simulink library "LopesDevelopmentLibrary"  (R2015b)
settings: Solver=ode45  StartTime=0.0  StopTime=10.0  RelTol=1e-3
values from neighbouring files (symbols this model uses):
  d2r = @(d) d*(pi/180)    [LopesDevelopmentLibrary_LoadParameters.m]
  ts = LopesParams.ts    [LopesDevelopmentLibrary_LoadParameters.m]
undefined symbols (not defined in the file or in its folder): anyParameterChanged, DiscIntNeverNeededParam, gcbh, LAP, LHF, LKF, LopesParams, macaddr, mxpcnetworkconfig, mxpcrtudprx, mxpcrtudptx, patientParametersChanged, port, PX, PZ, RAP, RHF, RKF, SelectorLOPESInSize, StrideTime_s, Time
undefined symbols (not defined in the file): LopesParamsSendDataArrayLen
libraries: LopesDevelopmentLibrary x327, simulink x100, dspmtrx3 x49, xpciplib x6, xpcnetworkbufferlib x5, dspsigops x4, dspstat3 x3, xpcethernetlib x2, visionstatistics x2, xpcseriallib x2, LopesDevelopmentLibraryTest x1, nmc x1
(part 8 of 12)

== system LopesDevelopmentLibrary/BlocksForInternalUse/GaitGeneration/CalculateReferenceGait/CalculateAbductionLeft ==
  note: This version of the CalculateAbduction calculates
      | the derivatives analytically. At the end of the script there is a (commented)
      | Matlab script that calculates the derivatives using the symbolic toolbox. It shows analytically that
      | the velocity is calculated correctly, and the acceleration is too complex to solve for.
      | For the acceleration, I put in random numbers as input and compared the result of my own (optimized) equation
      | and the equation found by Matla Symbolic toolbox. They are equal, so that proves that my equations are all okay.
  note: This block calculates the abduction angle for one leg, given the actual pelvis position and the desired ankle position.
      | It does not take into account rotations of the pelvis, but the deviations from that are so small that that is not a problem.
  Parameters : Inport
  PelvisTZ : Inport  Port=2
  AnkleTZ : Inport  Port=3
  xHF : Inport  Port=4
  xKF : Inport  Port=5
  Bus Selector : BusSelector  OutputSignals=Patient.PelvisWidth_m,Patient.UpperLegLength_m,Patient.LowerLegLength_m
  Demux{,1..3} (4 alike) : Demux  Outputs=3
  MATLAB Function : MATLAB Function  TreatAsAtomicUnit=on
  Signal Conversion : SignalConversion
  isRight : Constant  Value=isRight
  Abduction : Outport
  dAbduction_dx : Outport  Port=2
  d2Abduction_dx2 : Outport  Port=3
  wires:
  isRight/1 -> MATLAB Function/1(isRight)
  PelvisTZ/1 -> Demux/1
  AnkleTZ/1 -> Demux1/1
  xHF/1 -> Demux2/1
  xKF/1 -> Demux3/1
  Parameters/1 -> Bus Selector/1
  Bus Selector/1 -> MATLAB Function/14(w_pelvis)  "<PelvisWidth_m>"
  Bus Selector/2 -> MATLAB Function/15(l_upper)  "<UpperLegLength_m>"
  Bus Selector/3 -> MATLAB Function/16(l_lower)  "<LowerLegLength_m>"
  MATLAB Function/1(Abduction) -> Signal Conversion/1
  MATLAB Function/2(dAbductiondx) -> dAbduction_dx/1
  MATLAB Function/3(ddAbductiondx) -> d2Abduction_dx2/1
  Signal Conversion/1 -> Abduction/1
  Demux/2 -> MATLAB Function/3(dPelvisTZdx)
  Demux/3 -> MATLAB Function/4(ddPelvisTZdx)
  Demux/1 -> MATLAB Function/2(PelvisTZ)
  Demux1/2 -> MATLAB Function/6(dAnkleTZdx)
  Demux1/1 -> MATLAB Function/5(AnkleTZ)
  Demux1/3 -> MATLAB Function/7(ddAnkleTZdx)
  Demux2/2 -> MATLAB Function/9(dxHFdx)
  Demux2/3 -> MATLAB Function/10(ddxHFdx)
  Demux2/1 -> MATLAB Function/8(xHF)
  Demux3/3 -> MATLAB Function/13(ddxKFdx)
  Demux3/1 -> MATLAB Function/11(xKF)
  Demux3/2 -> MATLAB Function/12(dxKFdx)

== system LopesDevelopmentLibrary/BlocksForInternalUse/GaitGeneration/CalculateReferenceGait/CalculateAbductionRight ==
  note: This block calculates the abduction angle for one leg, given the actual pelvis position and the desired ankle position.
      | It does not take into account rotations of the pelvis, but the deviations from that are so small that that is not a problem.
  note: This version of the CalculateAbduction calculates
      | the derivatives analytically. At the end of the script there is a (commented)
      | Matlab script that calculates the derivatives using the symbolic toolbox. It shows analytically that
      | the velocity is calculated correctly, and the acceleration is too complex to solve for.
      | For the acceleration, I put in random numbers as input and compared the result of my own (optimized) equation
      | and the equation found by Matla Symbolic toolbox. They are equal, so that proves that my equations are all okay.
  Parameters : Inport
  PelvisTZ : Inport  Port=2
  AnkleTZ : Inport  Port=3
  xHF : Inport  Port=4
  xKF : Inport  Port=5
  Bus Selector : BusSelector  OutputSignals=Patient.PelvisWidth_m,Patient.UpperLegLength_m,Patient.LowerLegLength_m
  Demux{,1..3} (4 alike) : Demux  Outputs=3
  MATLAB Function : MATLAB Function  TreatAsAtomicUnit=on
  Signal Conversion : SignalConversion
  isRight : Constant  Value=isRight
  Abduction : Outport
  dAbduction_dx : Outport  Port=2
  d2Abduction_dx2 : Outport  Port=3
  wires:
  Demux3/2 -> MATLAB Function/12(dxKFdx)
  Demux3/1 -> MATLAB Function/11(xKF)
  Demux3/3 -> MATLAB Function/13(ddxKFdx)
  Demux2/1 -> MATLAB Function/8(xHF)
  Demux2/3 -> MATLAB Function/10(ddxHFdx)
  Demux2/2 -> MATLAB Function/9(dxHFdx)
  Demux1/3 -> MATLAB Function/7(ddAnkleTZdx)
  Demux1/1 -> MATLAB Function/5(AnkleTZ)
  Demux1/2 -> MATLAB Function/6(dAnkleTZdx)
  Demux/1 -> MATLAB Function/2(PelvisTZ)
  Demux/3 -> MATLAB Function/4(ddPelvisTZdx)
  Demux/2 -> MATLAB Function/3(dPelvisTZdx)
  Signal Conversion/1 -> Abduction/1
  MATLAB Function/3(ddAbductiondx) -> d2Abduction_dx2/1
  MATLAB Function/2(dAbductiondx) -> dAbduction_dx/1
  MATLAB Function/1(Abduction) -> Signal Conversion/1
  Bus Selector/3 -> MATLAB Function/16(l_lower)  "<LowerLegLength_m>"
  Bus Selector/2 -> MATLAB Function/15(l_upper)  "<UpperLegLength_m>"
  Bus Selector/1 -> MATLAB Function/14(w_pelvis)  "<PelvisWidth_m>"
  Parameters/1 -> Bus Selector/1
  xKF/1 -> Demux3/1
  xHF/1 -> Demux2/1
  AnkleTZ/1 -> Demux1/1
  PelvisTZ/1 -> Demux/1
  isRight/1 -> MATLAB Function/1(isRight)

== system LopesDevelopmentLibrary/BlocksForInternalUse/GaitGeneration/CalculateReferenceGait/FirstDerivativeWrtTime ==
  dydx : Inport
  dtdx : Inport  Port=2
  Divide : Product  Inputs=*/
  dydt : Outport
  wires:
  Divide/1 -> dydt/1
  dydx/1 -> Divide/1
  dtdx/1 -> Divide/2

== system LopesDevelopmentLibrary/BlocksForInternalUse/GaitGeneration/CalculateReferenceGait/SecondDerivativeWrtTime ==
  ddydx : Inport
  dtdx : Inport  Port=2
  Divide1 : Product  Inputs=*/
  Math Function : Math  Operator=square  SaturateOnIntegerOverflow=on
  ddydt : Outport
  wires:
  dtdx/1 -> Math Function/1
  Math Function/1 -> Divide1/2
  ddydx/1 -> Divide1/1
  Divide1/1 -> ddydt/1

== system LopesDevelopmentLibrary/BlocksForInternalUse/GaitGeneration/CalculateReferenceGait/Unactuated DOFS ==

== system LopesDevelopmentLibrary/BlocksForInternalUse/GaitGenerationStartStop/ExtraKeyPoints /LeftAnklePF ==
  parameters : Inport
  SetVelocity : Inport  Port=2
  Bus Creator4 : BusCreator  Inputs=2
  Bus Selector : BusSelector  OutputSignals=General.WalkingVelocity_m_s,Patient.BodyLength_m
  RegressionData : Constant  Value=LopesParams.GaitDataStartLeft.LAP
  RegressionData2KeyEvents : LopesDevelopmentLibrary/BlocksForInternalUse/GaitGeneration/RegressionData2KeyEvents
  Switch : Switch  Criteria=u2 > Threshold
  KeyEvents : Outport
  wires:
  Switch/1 -> Bus Creator4/1  "WalkingVelocity_m_s"
  SetVelocity/1 -> Switch/1, Switch/2
  Bus Selector/1 -> Switch/3  "<WalkingVelocity_m_s>"
  Bus Selector/2 -> Bus Creator4/2  "<BodyLength_m>"
  Bus Creator4/1 -> RegressionData2KeyEvents/2
  parameters/1 -> Bus Selector/1
  RegressionData/1 -> RegressionData2KeyEvents/1
  RegressionData2KeyEvents/1 -> KeyEvents/1

== system LopesDevelopmentLibrary/BlocksForInternalUse/GaitGenerationStartStop/ExtraKeyPoints /LeftHipFlexion ==
  parameters : Inport
  SetVelocity : Inport  Port=2
  Bus Creator4 : BusCreator  Inputs=2
  Bus Selector : BusSelector  OutputSignals=General.WalkingVelocity_m_s,Patient.BodyLength_m
  RegressionData : Constant  Value=LopesParams.GaitDataStartLeft.LHF
  RegressionData2KeyEvents : LopesDevelopmentLibrary/BlocksForInternalUse/GaitGeneration/RegressionData2KeyEvents
  Switch : Switch  Criteria=u2 > Threshold
  KeyEvents : Outport
  wires:
  RegressionData2KeyEvents/1 -> KeyEvents/1
  parameters/1 -> Bus Selector/1
  RegressionData/1 -> RegressionData2KeyEvents/1
  Bus Creator4/1 -> RegressionData2KeyEvents/2
  Bus Selector/2 -> Bus Creator4/2  "<BodyLength_m>"
  Bus Selector/1 -> Switch/3  "<WalkingVelocity_m_s>"
  SetVelocity/1 -> Switch/2, Switch/1
  Switch/1 -> Bus Creator4/1  "WalkingVelocity_m_s"

== system LopesDevelopmentLibrary/BlocksForInternalUse/GaitGenerationStartStop/ExtraKeyPoints /LeftKneeFlexion ==
  parameters : Inport
  SetVelocity : Inport  Port=2
  Bus Creator4 : BusCreator  Inputs=2
  Bus Selector : BusSelector  OutputSignals=General.WalkingVelocity_m_s,Patient.BodyLength_m
  RegressionData : Constant  Value=LopesParams.GaitDataStartLeft.LKF
  RegressionData2KeyEvents : LopesDevelopmentLibrary/BlocksForInternalUse/GaitGeneration/RegressionData2KeyEvents
  Switch : Switch  Criteria=u2 > Threshold
  KeyEvents : Outport
  wires:
  RegressionData2KeyEvents/1 -> KeyEvents/1
  RegressionData/1 -> RegressionData2KeyEvents/1
  parameters/1 -> Bus Selector/1
  Bus Creator4/1 -> RegressionData2KeyEvents/2
  Bus Selector/2 -> Bus Creator4/2  "<BodyLength_m>"
  Bus Selector/1 -> Switch/3  "<WalkingVelocity_m_s>"
  SetVelocity/1 -> Switch/2, Switch/1
  Switch/1 -> Bus Creator4/1  "WalkingVelocity_m_s"

== system LopesDevelopmentLibrary/BlocksForInternalUse/GaitGenerationStartStop/ExtraKeyPoints /PelvisTPX ==
  parameters : Inport
  SetVelocity : Inport  Port=2
  Bus Creator4 : BusCreator  Inputs=2
  Bus Selector : BusSelector  OutputSignals=General.WalkingVelocity_m_s,Patient.BodyLength_m
  RegressionData : Constant  Value=LopesParams.GaitDataStartLeft.PX
  RegressionData2KeyEvents : LopesDevelopmentLibrary/BlocksForInternalUse/GaitGeneration/RegressionData2KeyEvents
  Switch : Switch  Criteria=u2 > Threshold
  KeyEvents : Outport
  wires:
  Switch/1 -> Bus Creator4/1  "WalkingVelocity_m_s"
  SetVelocity/1 -> Switch/1, Switch/2
  Bus Selector/1 -> Switch/3  "<WalkingVelocity_m_s>"
  Bus Selector/2 -> Bus Creator4/2  "<BodyLength_m>"
  Bus Creator4/1 -> RegressionData2KeyEvents/2
  RegressionData/1 -> RegressionData2KeyEvents/1
  parameters/1 -> Bus Selector/1
  RegressionData2KeyEvents/1 -> KeyEvents/1

== system LopesDevelopmentLibrary/BlocksForInternalUse/GaitGenerationStartStop/ExtraKeyPoints /PelvisTPZ ==
  parameters : Inport
  SetVelocity : Inport  Port=2
  Bus Creator4 : BusCreator  Inputs=2
  Bus Selector : BusSelector  OutputSignals=General.WalkingVelocity_m_s,Patient.BodyLength_m
  RegressionData : Constant  Value=LopesParams.GaitDataStartLeft.PZ
  RegressionData2KeyEvents : LopesDevelopmentLibrary/BlocksForInternalUse/GaitGeneration/RegressionData2KeyEvents
  Switch : Switch  Criteria=u2 > Threshold
  KeyEvents : Outport
  wires:
  Switch/1 -> Bus Creator4/1  "WalkingVelocity_m_s"
  SetVelocity/1 -> Switch/1, Switch/2
  Bus Selector/1 -> Switch/3  "<WalkingVelocity_m_s>"
  Bus Selector/2 -> Bus Creator4/2  "<BodyLength_m>"
  Bus Creator4/1 -> RegressionData2KeyEvents/2
  RegressionData/1 -> RegressionData2KeyEvents/1
  parameters/1 -> Bus Selector/1
  RegressionData2KeyEvents/1 -> KeyEvents/1

== system LopesDevelopmentLibrary/BlocksForInternalUse/GaitGenerationStartStop/ExtraKeyPoints /RightAnklePF ==
  parameters : Inport
  SetVelocity : Inport  Port=2
  Bus Creator4 : BusCreator  Inputs=2
  Bus Selector : BusSelector  OutputSignals=General.WalkingVelocity_m_s,Patient.BodyLength_m
  RegressionData : Constant  Value=LopesParams.GaitDataStartLeft.RAP
  RegressionData2KeyEvents : LopesDevelopmentLibrary/BlocksForInternalUse/GaitGeneration/RegressionData2KeyEvents
  Switch : Switch  Criteria=u2 > Threshold
  KeyEvents : Outport
  wires:
  Switch/1 -> Bus Creator4/1  "WalkingVelocity_m_s"
  SetVelocity/1 -> Switch/1, Switch/2
  Bus Selector/1 -> Switch/3  "<WalkingVelocity_m_s>"
  Bus Selector/2 -> Bus Creator4/2  "<BodyLength_m>"
  Bus Creator4/1 -> RegressionData2KeyEvents/2
  parameters/1 -> Bus Selector/1
  RegressionData/1 -> RegressionData2KeyEvents/1
  RegressionData2KeyEvents/1 -> KeyEvents/1

== system LopesDevelopmentLibrary/BlocksForInternalUse/GaitGenerationStartStop/ExtraKeyPoints /RightHipFlexion ==
  parameters : Inport
  SetVelocity : Inport  Port=2
  Bus Creator4 : BusCreator  Inputs=2
  Bus Selector : BusSelector  OutputSignals=General.WalkingVelocity_m_s,Patient.BodyLength_m
  RegressionData : Constant  Value=LopesParams.GaitDataStartLeft.RHF
  RegressionData2KeyEvents : LopesDevelopmentLibrary/BlocksForInternalUse/GaitGeneration/RegressionData2KeyEvents
  Switch : Switch  Criteria=u2 > Threshold
  KeyEvents : Outport
  wires:
  RegressionData/1 -> RegressionData2KeyEvents/1
  RegressionData2KeyEvents/1 -> KeyEvents/1
  parameters/1 -> Bus Selector/1
  Bus Creator4/1 -> RegressionData2KeyEvents/2
  Bus Selector/2 -> Bus Creator4/2  "<BodyLength_m>"
  Bus Selector/1 -> Switch/3  "<WalkingVelocity_m_s>"
  SetVelocity/1 -> Switch/2, Switch/1
  Switch/1 -> Bus Creator4/1  "WalkingVelocity_m_s"

== system LopesDevelopmentLibrary/BlocksForInternalUse/GaitGenerationStartStop/ExtraKeyPoints /RightKneeFlexion ==
  parameters : Inport
  SetVelocity : Inport  Port=2
  Bus Creator4 : BusCreator  Inputs=2
  Bus Selector : BusSelector  OutputSignals=General.WalkingVelocity_m_s,Patient.BodyLength_m
  RegressionData : Constant  Value=LopesParams.GaitDataStartLeft.RKF
  RegressionData2KeyEvents : LopesDevelopmentLibrary/BlocksForInternalUse/GaitGeneration/RegressionData2KeyEvents
  Switch : Switch  Criteria=u2 > Threshold
  KeyEvents : Outport
  wires:
  RegressionData2KeyEvents/1 -> KeyEvents/1
  RegressionData/1 -> RegressionData2KeyEvents/1
  parameters/1 -> Bus Selector/1
  Bus Creator4/1 -> RegressionData2KeyEvents/2
  Bus Selector/2 -> Bus Creator4/2  "<BodyLength_m>"
  Bus Selector/1 -> Switch/3  "<WalkingVelocity_m_s>"
  SetVelocity/1 -> Switch/2, Switch/1
  Switch/1 -> Bus Creator4/1  "WalkingVelocity_m_s"

== system LopesDevelopmentLibrary/BlocksForInternalUse/LLC Communication/LLC Network Configuration/Variant Network Init ==
  note: 1) Only subsystems can be added as variant choices at this level
      | 2) Blocks cannot be connected at this level as connectivity is
      | automatically determined at simulation, based on the active variant
  note: I did not remove the inputs/outputs because that makes Matlab fail...
  Dummy_in : Inport
  Init_NonRT_UDP : Subsystem  VariantControl=LopesVariant_Non_RT
  Init_RT_2012b : Subsystem  VariantControl=LopesVariant_RT_2012b
  Init_RT_2014b : Subsystem  VariantControl=LopesVariant_RT_2014b
  Init_RT_2015b : Subsystem  VariantControl=LopesVariant_RT_2015b
  Dummy_out : Outport

== system LopesDevelopmentLibrary/BlocksForInternalUse/LLC Communication/LLCReceiveUDP/Debug ==

== system LopesDevelopmentLibrary/BlocksForInternalUse/LLC Communication/LLCReceiveUDP/UDPReceiveVariantChannel ==
  note: 1) Add Subsystem or Model blocks as valid variant choices.
      | 2) You cannot connect blocks at this level. At simulation, connectivity is automatically
      | determined, based on the active variant and port name matching.
  Dummy_in : Inport
  Receive_Non_RT : Subsystem  VariantControl=LopesVariant_Non_RT
  Receive_RT_2015b : Subsystem  VariantControl=LopesVariant_RT_2015b
  Receive_RT_R2012b : Subsystem  VariantControl=LopesVariant_RT_2012b
  Receive_RT_R2014b : Subsystem  VariantControl=LopesVariant_RT_2014b
  RecvData : Outport
  RecvLen : Outport  Port=2

== system LopesDevelopmentLibrary/BlocksForInternalUse/LLC Communication/LLCSendUDP/Debug ==

== system LopesDevelopmentLibrary/BlocksForInternalUse/LLC Communication/LLCSendUDP/UDPSendVariant ==
  Data : Inport
  Len : Inport  Port=2
  Enable : EnablePort
  Terminator : Terminator
  UDPSendVariantChannel : Subsystem  Variant=on
  wires:
  Data/1 -> UDPSendVariantChannel/1(SendData)
  Len/1 -> UDPSendVariantChannel/2(SendLen)
  UDPSendVariantChannel/1(Dummy_out) -> Terminator/1

== system LopesDevelopmentLibrary/BlocksForInternalUse/LLC Communication/UDP_Blocks/Network Configuration_RT_2012b  ==
  "ARP Init " : S-Function  Priority=0  FunctionName=xpcdebugarpinit  Parameters=Stats, Interface, IpAddress, SubnetMask, Gateway, EthernetId, Flags, BlockId, Retry, Timeout, Expiration, StaticAddressListIp, StaticAddressListMac, DiscoveryList, MulticastList, SampleTime  SFunctionDeploymentMode=off  EnableBusSupport=off  mask(arpinit){Interface=0, IpAddress=IpAddress, SubnetMask=SubnetMask, Gateway=Gateway, EthernetId=1, BlockId=0, SampleTime=-1, Flags=hex2dec('00000697'), Stats=off, Retry=5, Timeout=20, Expiration=20*60, StaticAddressListIp=[], StaticAddressListMac=[], DiscoveryList=[], MulticastList=[]}
      mask prompts: IpAddress "IP Address"; SubnetMask "Subnet Mask"; EthernetId "Ethernet ID"; BlockId "Block ID"; SampleTime "Sample Time"; Stats "Statistics Port"; StaticAddressListIp "[Static IP]"; StaticAddressListMac "[Static MAC]"; DiscoveryList "[Discovery IP]"; MulticastList "[Multicast IP]"
      mask help: ARP Init
      mask init:
      | xpclinklib('xpciplib');
      mask Help: web('arpdebug.htm',  '-helpbrowser');
      mask Display: disp('ARP Init');
  "Buffer Mngmt " : S-Function  Priority=-1  FunctionName=xpcnb  Parameters=pool_sizes, SampleTime, ShowTune  SFunctionDeploymentMode=off  EnableBusSupport=off  mask(xpcnbinit){SampleTime=-1, PoolSizes=[100 10 10 200], ShowTune=off}
      mask prompts: SampleTime "Sample time:"; PoolSizes "Buffer pool sizes (256, 512, 1024, 2048):"; ShowTune "Display tuning information"
      mask help: Network Buffer Initialization
      mask init:
      | [MaskDisplay, pool_sizes] = mxpcnbinit(2, PoolSizes);
      | 
      | set_param(gcb, 'MaskDisplay', MaskDisplay);
      mask Help: eval('xpcdoc(''NB_Init'')');
      mask Display: disp('Network Buffer\nManagement');
  "Ethernet Init " : S-Function  Priority=-1  FunctionName=xpcetherinit  Parameters="ID, Driver, Bus, Slot, VendorID, DeviceID, AddressSource, mac, TxSA, RxPromiscuous, RxBad, RxShort, MaxMTU, TxThreshold, TxBuffers, RxBuffers, ShowTune, numMulti, multicast,   NumRxBlks, SampleTime"  SFunctionDeploymentMode=off  EnableBusSupport=off  mask(xpcetherinit){ID=1, Driver=EthDrv, Bus=PciBus, Slot=PciSlot, SampleTime=-1, AddressSource=EEPROM, MAC=macaddr('00:00:00:00:00:00'), TxSA=off, RxPromiscuous=off, Multicast={}, RxBad=off, RxShort=off, MaxMTU=1518, TxThreshold=224, TxBuffers=128, RxBuffers=64, ShowTune=off, NumRxBlks=1}
      mask prompts: ID "Device ID:"; Bus "PCI bus:"; Slot "PCI slot:"; SampleTime "Sample time:"; AddressSource "Address source:"; TxSA "Tx source address from model"; RxPromiscuous "Rx promiscuous"; Multicast "Multicast address list:"; RxBad "Rx bad frames"; RxShort "Rx short frames"; MaxMTU "Max MTU:"; TxThreshold "Tx threshold:"; TxBuffers "Tx buffers:"; RxBuffers "Rx buffers:"; ShowTune "Display tuning information"; NumRxBlks "num rx blocks"
      mask help: Ethernet Initialization
      mask init:
      | VendorID = -1;
      | DeviceID = -1;
      | 
      | [MaskDisplay, VendorID, DeviceID, mac, numMulti, multicast] = mxpcetherinit(2, ID, Driver, Bus, Slot, MAC, Multicast);
      | 
      | set_param(gcb, 'MaskDisplay', MaskDisplay);
      mask Help: eval('xpcdoc(''Ether_Init'')');
      mask TypeOptions ID: 1 | 2 | 3 | 4 | 5 | 6 | 7 | 8
      mask TypeOptions AddressSource: EEPROM | Specify
      mask Callback AddressSource:
      | enables = get_param(gcb, 'MaskVisibilities');
      | if strcmp('Specify', get_param(gcb, 'AddressSource'))
      |     enables{strmatch('MAC',fieldnames(get_param(gcb,'DialogParameters')))} = 'on';
      | else
      |     enables{strmatch('MAC',fieldnames(get_param(gcb,'DialogParameters')))} = 'off';
      | end
      | set_param(gcb, 'MaskVisibilities', enables);
      mask Display: disp('Ethernet\nInitialization\nbus: 1 slot: 0\nId: 1\nIntel Gigabit');
  "IP Init " : S-Function  Priority=1  FunctionName=xpcdebugipinit  Parameters=Stats, Group, ArpId, IpAddress, SubnetMask, DefaultGateway, DefaultInterface, Flags, ToS, StartingId, TTL, SampleTime  SFunctionDeploymentMode=off  EnableBusSupport=off  mask(ipinit){Group=0, ArpId=[0], IpAddress=[IpAddress], SubnetMask=[SubnetMask], DefaultGateway=Gateway, DefaultInterface=0, SampleTime=-1, Flags=hex2dec('00000005'), ToS=hex2dec('00'), StartingId=10000, TTL=64, Stats=off}
      mask prompts: ArpId "[ARP ID]"; IpAddress "[IP Address]"; SubnetMask "[Subnet Mask]"; DefaultGateway "Default Gateway"; DefaultInterface "Default Interface"; SampleTime "Sample Time"; StartingId "Starting Id"; Stats "Statistics Port"
      mask help: IP Init
      mask init:
      | xpclinklib('xpciplib');
      mask Help: web('ipdebug.htm',  '-helpbrowser');
      mask Display: disp('IP Init');
  "UDP Init " : S-Function  Priority=2  FunctionName=xpcdebugudpinit  Parameters=Stats, Group, StartingPort, Flags, SampleTime  SFunctionDeploymentMode=off  EnableBusSupport=off  mask(udpinit){Group=0, StartingPort=10000, Flags=hex2dec('00000001'), SampleTime=-1, Stats=off}
      mask prompts: StartingPort "Starting Port"; SampleTime "Sample Time"; Stats "Statistics Port"
      mask help: UDP Init
      mask init:
      | xpclinklib('xpciplib');
      mask Help: web('udpdebug.htm',  '-helpbrowser');
      mask Display: disp('UDP Init');

== system LopesDevelopmentLibrary/BlocksForInternalUse/LLC Communication/UDP_Blocks/Network Configuration_RT_2014b  ==
  "ARP Init " : S-Function  Priority=0  FunctionName=xpcdebugarpinit  Parameters=Stats, Interface, IpAddress, SubnetMask, Gateway, EthernetId, Flags, BlockId, Retry, Timeout, Expiration, StaticAddressListIp, StaticAddressListMac, DiscoveryList, MulticastList, SampleTime  SFunctionDeploymentMode=off  EnableBusSupport=off  mask(arpinit){Interface=udpID, IpAddress=IpAddress, SubnetMask=SubnetMask, Gateway=Gateway, EthernetId=ID, BlockId=0, SampleTime=-1, Flags=hex2dec('00000697'), Stats=off, Retry=5, Timeout=20, Expiration=20*60, StaticAddressListIp=[], StaticAddressListMac=[], DiscoveryList=[], MulticastList=[]}
      mask prompts: IpAddress "IP Address"; SubnetMask "Subnet Mask"; EthernetId "Ethernet ID"; BlockId "Block ID"; SampleTime "Sample Time"; Stats "Statistics Port"; StaticAddressListIp "[Static IP]"; StaticAddressListMac "[Static MAC]"; DiscoveryList "[Discovery IP]"; MulticastList "[Multicast IP]"
      mask help: ARP Init
      mask init:
      | xpclinklib('xpciplib');
      mask Help: web('arpdebug.htm',  '-helpbrowser');
      mask Display: disp('ARP Init');
  "Buffer Mngmt " : xpcnetworkbufferlib/Buffer Mngmt   Priority=-1  SampleTime=-1  PoolSizes=[100 10 10 200]  ShowTune=off
  "Ethernet Init " : xpcethernetlib/Ethernet Init   Priority=-1  ID=1  Driver=Intel Gigabit  Bus=PciBus  Slot=PciSlot  SampleTime=-1  AddressSource=EEPROM  MAC=macaddr('00:00:00:00:00:00')  TxSA=off  RxPromiscuous=off  Multicast={}  RxBad=off  RxShort=off  MaxMTU=1518  TxThreshold=224  TxBuffers=128  RxBuffers=64  ShowTune=off  NumRxBlks=1
  "IP Init " : S-Function  Priority=1  FunctionName=xpcdebugipinit  Parameters=Stats, Group, ArpId, IpAddress, SubnetMask, DefaultGateway, DefaultInterface, Flags, ToS, StartingId, TTL, SampleTime  SFunctionDeploymentMode=off  EnableBusSupport=off  mask(ipinit){Group=udpID, ArpId=[udpID], IpAddress=[IpAddress], SubnetMask=[SubnetMask], DefaultGateway=Gateway, DefaultInterface=0, SampleTime=-1, Flags=hex2dec('00000005'), ToS=hex2dec('00'), StartingId=10000, TTL=64, Stats=off}
      mask prompts: ArpId "[ARP ID]"; IpAddress "[IP Address]"; SubnetMask "[Subnet Mask]"; DefaultGateway "Default Gateway"; DefaultInterface "Default Interface"; SampleTime "Sample Time"; StartingId "Starting Id"; Stats "Statistics Port"
      mask help: IP Init
      mask init:
      | xpclinklib('xpciplib');
      mask Help: web('ipdebug.htm',  '-helpbrowser');
      mask Display: disp('IP Init');
  "UDP Init " : S-Function  Priority=2  FunctionName=xpcdebugudpinit  Parameters=Stats, Group, StartingPort, Flags, SampleTime  SFunctionDeploymentMode=off  EnableBusSupport=off  mask(udpinit){Group=udpID, StartingPort=10000, Flags=hex2dec('00000001'), SampleTime=-1, Stats=off}
      mask prompts: StartingPort "Starting Port"; SampleTime "Sample Time"; Stats "Statistics Port"
      mask help: UDP Init
      mask init:
      | xpclinklib('xpciplib');
      mask Help: web('udpdebug.htm',  '-helpbrowser');
      mask Display: disp('UDP Init');

== system LopesDevelopmentLibrary/BlocksForInternalUse/LLC Communication/UDP_Blocks/Network Configuration_RT_2015b ==
  "ARP Init " : S-Function  Priority=0  FunctionName=xpcdebugarpinit  Parameters=Stats, Interface, IpAddress, SubnetMask, Gateway, EthernetId, Flags, BlockId, Retry, Timeout, Expiration, StaticAddressListIp, StaticAddressListMac, DiscoveryList, MulticastList, SampleTime  SFunctionDeploymentMode=off  EnableBusSupport=off  mask(arpinit){Interface=udpID, IpAddress=IpAddress, SubnetMask=SubnetMask, Gateway=Gateway, EthernetId=ID, BlockId=0, SampleTime=-1, Flags=hex2dec('00000697'), Stats=off, Retry=5, Timeout=20, Expiration=20*60, StaticAddressListIp=[], StaticAddressListMac=[], DiscoveryList=[], MulticastList=MulticastList}
      mask prompts: IpAddress "IP Address"; SubnetMask "Subnet Mask"; EthernetId "Ethernet ID"; BlockId "Block ID"; SampleTime "Sample Time"; Stats "Statistics Port"; StaticAddressListIp "[Static IP]"; StaticAddressListMac "[Static MAC]"; DiscoveryList "[Discovery IP]"; MulticastList "[Multicast IP]"
      mask help: ARP Init
      mask init:
      | xpclinklib('xpciplib');
      mask Help: web('arpdebug.htm',  '-helpbrowser');
      mask Display: disp('ARP Init');
  "Buffer Mngmt " : xpcnetworkbufferlib/Buffer Mngmt   Priority=-1  SampleTime=-1  PoolSizes=[100 10 10 200]  ShowTune=off
  "Ethernet Init " : xpcethernetlib/Ethernet Init   Priority=-1  ID=1  Driver=Intel Gigabit  Bus=PciBus  Slot=PciSlot  SampleTime=-1  AddressSource=EEPROM  MAC=macaddr('00:00:00:00:00:00')  TxSA=off  RxPromiscuous=off  Multicast=Multicast  RxBad=off  RxShort=off  MaxMTU=1518  TxThreshold=224  TxBuffers=128  RxBuffers=64  ShowTune=off  NumRxBlks=1
  "IP Init " : S-Function  Priority=1  FunctionName=xpcdebugipinit  Parameters=Stats, Group, ArpId, IpAddress, SubnetMask, DefaultGateway, DefaultInterface, Flags, ToS, StartingId, TTL, SampleTime  SFunctionDeploymentMode=off  EnableBusSupport=off  mask(ipinit){Group=udpID, ArpId=[udpID], IpAddress=[IpAddress], SubnetMask=[SubnetMask], DefaultGateway=Gateway, DefaultInterface=0, SampleTime=-1, Flags=hex2dec('00000005'), ToS=hex2dec('00'), StartingId=10000, TTL=64, Stats=off}
      mask prompts: ArpId "[ARP ID]"; IpAddress "[IP Address]"; SubnetMask "[Subnet Mask]"; DefaultGateway "Default Gateway"; DefaultInterface "Default Interface"; SampleTime "Sample Time"; StartingId "Starting Id"; Stats "Statistics Port"
      mask help: IP Init
      mask init:
      | xpclinklib('xpciplib');
      mask Help: web('ipdebug.htm',  '-helpbrowser');
      mask Display: disp('IP Init');
  "UDP Init " : S-Function  Priority=2  FunctionName=xpcdebugudpinit  Parameters=Stats, Group, StartingPort, Flags, SampleTime  SFunctionDeploymentMode=off  EnableBusSupport=off  mask(udpinit){Group=udpID, StartingPort=10000, Flags=hex2dec('00000001'), SampleTime=-1, Stats=off}
      mask prompts: StartingPort "Starting Port"; SampleTime "Sample Time"; Stats "Statistics Port"
      mask help: UDP Init
      mask init:
      | xpclinklib('xpciplib');
      mask Help: web('udpdebug.htm',  '-helpbrowser');
      mask Display: disp('UDP Init');

== system LopesDevelopmentLibrary/BlocksForInternalUse/LLC Communication/UDP_Blocks/Receive_RT_2012b  ==
  "Buffer " : S-Function  FunctionName=xpcnbbuffer  Parameters=chainSize, bufferSize, Threshold  SFunctionDeploymentMode=off  EnableBusSupport=off  mask(xpcnbbuffer){ChainSize=1, BufferSize=0, Threshold=0}
      mask prompts: ChainSize "Chain size:"; BufferSize "Buffer size:"
      mask help:
      | Network Buffer Buffering
      |
      | Chain size = inf --> No buffering, all packets passed through
      | Chain size = 0   --> Deletes all packets, none passed through
      | Chain size > 0   --> Passes through first "Chain size" packets
      | Chain size < 0   --> Passes through last "Chain size" packets
      |
      | Buffer size = inf --> All remaining packets are buffered, none are deleted
      | Buffer size = 0   --> No buffering, deletes all remaining packets
      | Buffer size > 0   --> Buffers remaining first "Buffer size" packets
      | Buffer size < 0   --> Buffers remaining last "Buffer size" packets
      |
      | Threshold = 0 --> No threshold
      | Threshold > 0 --> Delay passing through packets till threshold is met once
      | Threshold < 0 --> Passes through packets if "Threshold" packets are buffered
      mask init:
      | [MaskDisplay, chainSize, bufferSize] = mxpcnbbuffer(2, ChainSize, BufferSize, Threshold);
      | 
      | set_param(gcb, 'MaskDisplay', MaskDisplay);
      mask Help: helpview(fullfile(docroot, 'mapfiles', 'xpc.map'), 'NB_Buffer')
      mask Display: disp('NB\nBuffering\n\n');port_label('output', 1, '1');
  "Extract " : S-Function  FunctionName=xpcnbextract  Parameters=packetSize  SFunctionDeploymentMode=off  EnableBusSupport=off  mask(xpcnbextract){PacketSize=Receive3}
      mask prompts: PacketSize "Packet size (-1: inherit):"
      mask help: Network Buffer Extract
      mask init:
      | [packetSize] = mxpcnbextract(2,PacketSize);
      mask Help: helpview(fullfile(docroot, 'mapfiles', 'xpc.map'), 'NB_Extract')
      mask Display: disp('NB Extract\n');port_label('output', 2, 'length');
  Terminator : Terminator
  "UDP Consume " : S-Function  FunctionName=xpcudpconsume  Parameters=Group, VectorSize, SampleTime  SFunctionDeploymentMode=off  EnableBusSupport=off  mask(udpconsume){Group=0, VectorSize=0, SampleTime=Receive4}
      mask prompts: Group "IP Group"; VectorSize "Output port width:"; SampleTime "Sample time:"
      mask help: UDP Consume
      mask Help: helpview(fullfile(docroot, 'mapfiles', 'xpc.map'), 'RT_UDP_CONSUME')
      mask Display:
      | if VectorSize
      |     disp('UDP Consume\n\n\n\n\n\n\n');
      |     port_label('output', 1, 'Buffers');
      |     port_label('output', 2, 'Source IP Address');
      |     port_label('output', 3, 'Destination IP Address');
      |     port_label('output', 4, 'Local UDP Port');
      |     port_label('output', 5, 'Remote UDP Port');
      |     port_label('output', 6, 'Chain Size');
      | else
      |     disp('UDP Consume');
      |     port_label('output', 1, 'Buffers');
      |     port_label('output', 2, 'Chain Size');
      | end
  "UDP Rx " : S-Function  Priority=5  FunctionName=xpcudprx  Parameters=Group, SourceAddress, sip, LocalPort, lup, SampleTime  SFunctionDeploymentMode=off  EnableBusSupport=off  mask(udprx){Group=0, sip=Any, SourceAddress=Receive1, lup=Specify, LocalPort=Receive2, SampleTime=Receive4}
      mask prompts: Group "IP Group"; sip "Source IP Address"; SourceAddress "IP address to receive from (0.0.0.0 for accepting all):"; lup "Local UDP Port"; LocalPort "IP port to receive from:"; SampleTime "Sample time:"
      mask help: UDP Rx
      mask init:
      | if SourceAddress == 0
      |     sip = 3;
      | end
      | 
      | SourceAddress = ipaddr(SourceAddress);
      mask Help: helpview(fullfile(docroot, 'mapfiles', 'xpc.map'), 'RT_UDP_RX')
      mask TypeOptions sip: Specify | Port | Any
      mask TypeOptions lup: Specify | Port | Any
      mask Display: disp('UDP Rx');
  Out1 : Outport  OutDataTypeStr=uint8
  Out2 : Outport  Port=2  OutDataTypeStr=double
  wires:
  "UDP Consume "/2 -> Terminator/1
  "UDP Consume "/1 -> "Extract "/1
  "UDP Rx "/1 -> "Buffer "/1
  "Buffer "/1 -> "UDP Consume "/1
  "Extract "/1 -> Out1/1
  "Extract "/2 -> Out2/1

== system LopesDevelopmentLibrary/BlocksForInternalUse/LLC Communication/UDP_Blocks/Receive_RT_2014b  ==
  "Buffer " : S-Function  FunctionName=xpcnbbuffer  Parameters=chainSize, bufferSize, Threshold  SFunctionDeploymentMode=off  EnableBusSupport=off  mask(xpcnbbuffer){ChainSize=1, BufferSize=0, Threshold=0}
      mask prompts: ChainSize "Chain size:"; BufferSize "Buffer size:"
      mask help:
      | Network Buffer Buffering
      |
      | Chain size = inf --> No buffering, all packets passed through
      | Chain size = 0   --> Deletes all packets, none passed through
      | Chain size > 0   --> Passes through first "Chain size" packets
      | Chain size < 0   --> Passes through last "Chain size" packets
      |
      | Buffer size = inf --> All remaining packets are buffered, none are deleted
      | Buffer size = 0   --> No buffering, deletes all remaining packets
      | Buffer size > 0   --> Buffers remaining first "Buffer size" packets
      | Buffer size < 0   --> Buffers remaining last "Buffer size" packets
      |
      | Threshold = 0 --> No threshold
      | Threshold > 0 --> Delay passing through packets till threshold is met once
      | Threshold < 0 --> Passes through packets if "Threshold" packets are buffered
      mask init:
      | [MaskDisplay, chainSize, bufferSize] = mxpcnbbuffer(2, ChainSize, BufferSize, Threshold);
      | 
      | set_param(gcb, 'MaskDisplay', MaskDisplay);
      mask Help: helpview(fullfile(docroot, 'mapfiles', 'xpc.map'), 'NB_Buffer')
      mask Display: disp('NB\nBuffering\n\n');port_label('output', 1, '1');
  "Extract " : S-Function  FunctionName=xpcnbextract  Parameters=packetSize  SFunctionDeploymentMode=off  EnableBusSupport=off  mask(xpcnbextract){PacketSize=Receive3}
      mask prompts: PacketSize "Packet size (-1: inherit):"
      mask help: Network Buffer Extract
      mask init:
      | [packetSize] = mxpcnbextract(2,PacketSize);
      mask Help: helpview(fullfile(docroot, 'mapfiles', 'xpc.map'), 'NB_Extract')
      mask Display: disp('NB Extract\n');port_label('output', 2, 'length');
  Terminator : Terminator
  "UDP Consume " : S-Function  FunctionName=xpcudpconsume  Parameters=Group, VectorSize, SampleTime  SFunctionDeploymentMode=off  EnableBusSupport=off  mask(udpconsume){Group=udpID, VectorSize=0, SampleTime=Receive4}
      mask prompts: Group "IP Group"; VectorSize "Output port width:"; SampleTime "Sample time:"
      mask help: UDP Consume
      mask Help: helpview(fullfile(docroot, 'mapfiles', 'xpc.map'), 'RT_UDP_CONSUME')
      mask Display:
      | if VectorSize
      |     disp('UDP Consume\n\n\n\n\n\n\n');
      |     port_label('output', 1, 'Buffers');
      |     port_label('output', 2, 'Source IP Address');
      |     port_label('output', 3, 'Destination IP Address');
      |     port_label('output', 4, 'Local UDP Port');
      |     port_label('output', 5, 'Remote UDP Port');
      |     port_label('output', 6, 'Chain Size');
      | else
      |     disp('UDP Consume');
      |     port_label('output', 1, 'Buffers');
      |     port_label('output', 2, 'Chain Size');
      | end
  "UDP Rx " : S-Function  Priority=5  FunctionName=xpcudprx  Parameters=Group, SourceAddress, sip, LocalPort, lup, SampleTime  SFunctionDeploymentMode=off  EnableBusSupport=off  mask(udprx){Group=udpID, sip=Any, SourceAddress=Receive1, lup=Specify, LocalPort=Receive2, SampleTime=Receive4}
      mask prompts: Group "IP Group"; sip "Source IP Address"; SourceAddress "IP address to receive from (0.0.0.0 for accepting all):"; lup "Local UDP Port"; LocalPort "IP port to receive from:"; SampleTime "Sample time:"
      mask help: UDP Rx
      mask init:
      | if SourceAddress == 0
      |     sip = 3;
      | else
      |     sip = 1;
      | end
      mask Help: helpview(fullfile(docroot, 'mapfiles', 'xpc.map'), 'RT_UDP_RX')
      mask TypeOptions sip: Specify | Port | Any
      mask TypeOptions lup: Specify | Port | Any
      mask Display: disp('UDP Rx');
  Out1 : Outport  OutDataTypeStr=uint8
  Out2 : Outport  Port=2  OutDataTypeStr=double
  wires:
  "UDP Consume "/2 -> Terminator/1
  "UDP Consume "/1 -> "Extract "/1
  "UDP Rx "/1 -> "Buffer "/1
  "Buffer "/1 -> "UDP Consume "/1
  "Extract "/1 -> Out1/1
  "Extract "/2 -> Out2/1

== system LopesDevelopmentLibrary/BlocksForInternalUse/LLC Communication/UDP_Blocks/Receive_RT_2015b ==
  Buffer 1 : xpcnetworkbufferlib/Manage   ChainSize=1  BufferSize=0  Threshold=0
  Extract 1 : xpcnetworkbufferlib/Extract   PacketSize=Receive3
  Terminator : Terminator
  UDP Consume 1 : xpciplib/UDP Consume   Group=udpID  VectorSize=0  SampleTime=Receive4
  UDP Rx 1 : xpciplib/UDP Rx   Priority=5  Group=udpID  sip=Any  SourceAddress=Receive1  lup=Specify  LocalPort=Receive2  SampleTime=Receive4
  Out1 : Outport  OutDataTypeStr=uint8
  Out2 : Outport  Port=2  OutDataTypeStr=double
  wires:
  UDP Consume 1/2 -> Terminator/1
  UDP Consume 1/1 -> Extract 1/1
  UDP Rx 1/1 -> Buffer 1/1
  Buffer 1/1 -> UDP Consume 1/1
  Extract 1/1 -> Out1/1
  Extract 1/2 -> Out2/1

== system LopesDevelopmentLibrary/BlocksForInternalUse/LLC Communication/UDP_Blocks/Send_RT_2012b ==
  In1 : Inport  OutDataTypeStr=uint8
  In2 : Inport  Port=2  OutDataTypeStr=double
  "Compose " : S-Function  FunctionName=xpcnbcompose  SFunctionDeploymentMode=off  EnableBusSupport=off  mask(xpcnbcompose){}
      mask help: Network Buffer Compose
      mask init:
      | mxpcnbcompose(2);
      mask Help: helpview(fullfile(docroot, 'mapfiles', 'xpc.map'), 'NB_Compose')
      mask Display: disp('NB Compose\n');port_label('input', 2, 'length');
  "UDP Produce " : S-Function  Priority=5  FunctionName=xpcudpproduce  Parameters=Group, SrcIp, sip, DstIp, dip, LocPort, lup, RemPort, rup, SampleTime  SFunctionDeploymentMode=off  EnableBusSupport=off  mask(udpproduce){Group=0, sip=Auto, SrcIp=0.0.0.0, dip=Specify, DstIp=Send1, rup=Specify, RemPort=Send2, lup=Auto, LocPort=Send3, SampleTime=Send4}
      mask prompts: Group "IP Group"; sip "Source IP Address"; SrcIp "Source IP Address"; dip "Destination IP Address"; DstIp "IP address to send to (255.255.255.255 for broadcast):"; rup "Remote UDP Port"; RemPort "Remote IP port to send to:"; lup "Local UDP Port"; LocPort "Use the following local IP port (-1 for automatic assignment):"; SampleTime "Sample time:"
      mask help: UDP Produce
      mask init:
      | if LocPort == -1
      |     lup = 3;
      | end
      | 
      | SrcIp = ipaddr(SrcIp);
      | DstIp = ipaddr(DstIp);
      mask Help: helpview(fullfile(docroot, 'mapfiles', 'xpc.map'), 'RT_UDP_PRODUCE')
      mask TypeOptions sip: Specify | Port | Auto
      mask TypeOptions dip: Specify | Port
      mask TypeOptions rup: Specify | Port
      mask TypeOptions lup: Specify | Port | Auto
      mask Display: disp('UDP Produce');
  "UDP Tx " : xpciplib/UDP Tx   Priority=5  Group=0  TTL=-1  ToS=-1  SampleTime=Send4
  wires:
  "UDP Produce "/1 -> "UDP Tx "/1
  "Compose "/1 -> "UDP Produce "/1
  In1/1 -> "Compose "/1
  In2/1 -> "Compose "/2

== system LopesDevelopmentLibrary/BlocksForInternalUse/LLC Communication/UDP_Blocks/Send_RT_2014b ==
  In1 : Inport  OutDataTypeStr=uint8
  In2 : Inport  Port=2  OutDataTypeStr=double
  "Compose " : S-Function  FunctionName=xpcnbcompose  SFunctionDeploymentMode=off  EnableBusSupport=off  mask(xpcnbcompose){}
      mask help: Network Buffer Compose
      mask init:
      | mxpcnbcompose(2);
      mask Help: helpview(fullfile(docroot, 'mapfiles', 'xpc.map'), 'NB_Compose')
      mask Display: disp('NB Compose\n');port_label('input', 2, 'length');
  "UDP Produce " : S-Function  Priority=5  FunctionName=xpcudpproduce  Parameters=Group, SrcIp, sip, DstIp, dip, LocPort, lup, RemPort, rup, SampleTime  SFunctionDeploymentMode=off  EnableBusSupport=off  mask(udpproduce){Group=udpID, sip=Auto, SrcIp=0.0.0.0, dip=Specify, DstIp=Send1, rup=Specify, RemPort=Send2, lup=Auto, LocPort=Send3, SampleTime=Send4}
      mask prompts: Group "IP Group"; sip "Source IP Address"; SrcIp "Source IP Address"; dip "Destination IP Address"; DstIp "IP address to send to (255.255.255.255 for broadcast):"; rup "Remote UDP Port"; RemPort "Remote IP port to send to:"; lup "Local UDP Port"; LocPort "Use the following local IP port (-1 for automatic assignment):"; SampleTime "Sample time:"
      mask help: UDP Produce
      mask init:
      | if LocPort == -1
      |     lup = 3;
      | else
      |     lup = 1;
      | end
      | 
      | SrcIp = ipaddr(SrcIp);
      | DstIp = ipaddr(DstIp);
      mask Help: helpview(fullfile(docroot, 'mapfiles', 'xpc.map'), 'RT_UDP_PRODUCE')
      mask TypeOptions sip: Specify | Port | Auto
      mask TypeOptions dip: Specify | Port
      mask TypeOptions rup: Specify | Port
      mask TypeOptions lup: Specify | Port | Auto
      mask Display: disp('UDP Produce');
  "UDP Tx " : xpciplib/UDP Tx   Priority=5  Group=udpID  TTL=-1  ToS=-1  SampleTime=Send4
  wires:
  "UDP Produce "/1 -> "UDP Tx "/1
  "Compose "/1 -> "UDP Produce "/1
  In1/1 -> "Compose "/1
  In2/1 -> "Compose "/2

== system LopesDevelopmentLibrary/BlocksForInternalUse/LLC Communication/UDP_Blocks/Send_RT_2015b ==
  In1 : Inport  OutDataTypeStr=uint8
  In2 : Inport  Port=2  OutDataTypeStr=double
  "Compose " : xpcnetworkbufferlib/Compose 
  "UDP Produce " : xpciplib/UDP Produce   Priority=5  Group=udpID  sip=Auto  SrcIp=0.0.0.0  dip=Specify  DstIp=Send1  rup=Specify  RemPort=Send2  lup=Auto  LocPort=Send3  SampleTime=Send4
  "UDP Tx " : xpciplib/UDP Tx   Priority=5  Group=udpID  TTL=-1  ToS=-1  SampleTime=Send4
  wires:
  "UDP Produce "/1 -> "UDP Tx "/1
  "Compose "/1 -> "UDP Produce "/1
  In1/1 -> "Compose "/1
  In2/1 -> "Compose "/2

== system LopesDevelopmentLibrary/GaitGeneration/CalculateBreaksCoefs/Calculate/ActuatedDOFS ==

== system LopesDevelopmentLibrary/GaitGeneration/CalculateBreaksCoefs/Calculate/GenerateFakeTime ==
  note: This block generates a 'fake time' signal: (a placeholder) and a
      | fake StrideTime. These are provided in order to be able to use block that
      | require the existence of these signals. By giving fake (i.e., wrong) values,
      | the calculations in those blocks involving these signals will be wrong, but these
      | calculations are never used, so this does not matter.
  Bus Creator13 : BusCreator  Inputs=2
  FakeBreaksTime : Constant  Value=[0,100]
  FakeCoefsTime : Constant  Value=[0,0,0;0,0,0]
  FakeStrideTime1 : Constant
  FakeStrideTime_s : Outport
  FakeTime : Outport  Port=2
  wires:
  FakeCoefsTime/1 -> Bus Creator13/2  "coefs"
  FakeBreaksTime/1 -> Bus Creator13/1  "breaks"
  Bus Creator13/1 -> FakeTime/1  "Time"
  FakeStrideTime1/1 -> FakeStrideTime_s/1

== system LopesDevelopmentLibrary/GaitGeneration/CalculateBreaksCoefs/Calculate/LeftAnklePlantarflexion1 ==
  parameters : Inport
  StepHeight_AnkleDorsiflexion_pct : Inport  Port=2
  Prepositioning_AnkleAngle_pct : Inport  Port=3
  Pushoff_Timing_pct : Inport  Port=4
  AnkleAnglePrepositioning : LopesDevelopmentLibrary/Various/AddToMatrixElement  row=3  col=2  minimum=d2r(-inf)  maximum=d2r(inf)
  AnkleAnglePrepositioning1 : LopesDevelopmentLibrary/Various/AddToMatrixElement  row=6  col=2  minimum=d2r(-inf)  maximum=d2r(inf)
  Gain : Gain  Gain=1/100*d2r(20)
  Gain1 : Gain  Gain=-1/100*d2r(5)
  RegressionData : Constant  Value=LopesParams.GaitData.LAP
  RegressionData2KeyEvents1 : LopesDevelopmentLibrary/BlocksForInternalUse/GaitGeneration/RegressionData2KeyEvents
  TimingPushoff : LopesDevelopmentLibrary/Various/AddToMatrixElement  row=4  col=1  minimum=d2r(-inf)  maximum=d2r(inf)
  KeyEvents : Outport
  wires:
  Prepositioning_AnkleAngle_pct/1 -> Gain/1
  AnkleAnglePrepositioning/1 -> TimingPushoff/1
  TimingPushoff/1 -> KeyEvents/1
  Pushoff_Timing_pct/1 -> TimingPushoff/2
  Gain/1 -> AnkleAnglePrepositioning/2
  RegressionData/1 -> RegressionData2KeyEvents1/1
  parameters/1 -> RegressionData2KeyEvents1/2
  RegressionData2KeyEvents1/1 -> AnkleAnglePrepositioning1/1
  AnkleAnglePrepositioning1/1 -> AnkleAnglePrepositioning/1
  Gain1/1 -> AnkleAnglePrepositioning1/2
  StepHeight_AnkleDorsiflexion_pct/1 -> Gain1/1

== system LopesDevelopmentLibrary/GaitGeneration/CalculateBreaksCoefs/Calculate/LeftAnkleZ1 ==
  note: Maximum of 15 cm extra circumduction
  parameters : Inport
  WeightShift_StepWidth_pct : Inport  Port=2
  Circumduction_CircumductionLeft_pct : Inport  Port=3
  AddToMatrixElement : LopesDevelopmentLibrary/Various/AddToMatrixElement  row=3  col=2  minimum=-inf  maximum=inf
  AssignMatrixElement : LopesDevelopmentLibrary/Various/AssignMatrixElement  row=3  col=2  minimum=-inf  maximum=inf
  Bias : Bias  Bias=1
  CircumductionGain : Gain  Gain=0.01*(-0.15)
  Gain2 : Gain  Gain=0.01
  K1toK3 : dspmtrx3/Submatrix  RowSpan=All rows  RowStartMode=Index  RowStartIndex=row  RowEndMode=Index  RowEndIndex=1  ColSpan=One column  ColStartMode=Index  ColStartIndex=2  ColEndMode=Last  ColEndIndex=1
  MinMax : MinMax
  MultiplyMatrixElement : LopesDevelopmentLibrary/Various/MultiplyMatrixElement  row=1  col=2  minimum=-inf  maximum=inf
  MultiplyMatrixElement1 : LopesDevelopmentLibrary/Various/MultiplyMatrixElement  row=2  col=2  minimum=-inf  maximum=inf
  RegressionData : Constant  Value=LopesParams.GaitData.LAnkleZ
  RegressionData2KeyEvents : LopesDevelopmentLibrary/BlocksForInternalUse/GaitGeneration/RegressionData2KeyEvents
  KeyEvents : Outport
  wires:
  RegressionData2KeyEvents/1 -> MultiplyMatrixElement/1
  RegressionData/1 -> RegressionData2KeyEvents/1
  parameters/1 -> RegressionData2KeyEvents/2
  WeightShift_StepWidth_pct/1 -> Gain2/1
  Gain2/1 -> Bias/1
  Bias/1 -> MultiplyMatrixElement/2, MultiplyMatrixElement1/2
  AddToMatrixElement/1 -> KeyEvents/1
  MultiplyMatrixElement/1 -> MultiplyMatrixElement1/1
  MultiplyMatrixElement1/1 -> K1toK3/1, AssignMatrixElement/1
  K1toK3/1 -> MinMax/1
  MinMax/1 -> AssignMatrixElement/2
  AssignMatrixElement/1 -> AddToMatrixElement/1
  Circumduction_CircumductionLeft_pct/1 -> CircumductionGain/1
  CircumductionGain/1 -> AddToMatrixElement/2

== system LopesDevelopmentLibrary/GaitGeneration/CalculateBreaksCoefs/Calculate/LeftHipFlexion1 ==
  parameters : Inport
  HipExtensionOffset_pct : Inport  Port=2
  Steplength_Length_pct : Inport  Port=3
  SteplengthOtherLeg_Length_pct : Inport  Port=4
  StepHeight_KneeFlexion_pct : Inport  Port=5
  AddToMatrixColumn : LopesDevelopmentLibrary/Various/AddToMatrixColumn  col=2  minimum=-inf  maximum=inf
  Bias : Bias  Bias=100
  Bias1 : Bias  Bias=100
  Gain1 : Gain  Gain=1/100
  Gain2 : Gain  Gain=1/100
  Gain3 : Gain  Gain=0.01* d2r(2.5)
  Gain4 : Gain  Gain=0.01* d2r(5)
  GainHipExtensionOffset : Gain  Gain=-0.01* d2r(10)
  KneeFlexionStepheight : LopesDevelopmentLibrary/Various/AddToMatrixElement  row=5  col=2  minimum=0  maximum=d2r(90)
  KneeFlexionStepheight1 : LopesDevelopmentLibrary/Various/AddToMatrixElement  row=6  col=2  minimum=0  maximum=d2r(90)
  MultiplyMatrixElement : LopesDevelopmentLibrary/Various/MultiplyMatrixElement  row=6  col=2  minimum=-inf  maximum=inf
  MultiplyMatrixElement1 : LopesDevelopmentLibrary/Various/MultiplyMatrixElement  row=4  col=2  minimum=-inf  maximum=inf
  MultiplyMatrixElement2 : LopesDevelopmentLibrary/Various/MultiplyMatrixElement  row=1  col=2  minimum=-inf  maximum=inf
  MultiplyMatrixElement3 : LopesDevelopmentLibrary/Various/MultiplyMatrixElement  row=2  col=2  minimum=-inf  maximum=inf
  RatioFlexionExtension : Gain
  RegressionData : Constant  Value=LopesParams.GaitData.LHF
  RegressionData2KeyEvents : LopesDevelopmentLibrary/BlocksForInternalUse/GaitGeneration/RegressionData2KeyEvents
  KeyEvents : Outport
  wires:
  MultiplyMatrixElement1/1 -> KeyEvents/1
  AddToMatrixColumn/1 -> MultiplyMatrixElement/1
  Gain2/1 -> MultiplyMatrixElement1/2
  Steplength_Length_pct/1 -> Bias/1
  Bias/1 -> Gain1/1
  Gain1/1 -> MultiplyMatrixElement3/2, MultiplyMatrixElement2/2, MultiplyMatrixElement/2
  Bias1/1 -> Gain2/1
  SteplengthOtherLeg_Length_pct/1 -> RatioFlexionExtension/1
  RegressionData/1 -> RegressionData2KeyEvents/1
  parameters/1 -> RegressionData2KeyEvents/2
  KneeFlexionStepheight/1 -> KneeFlexionStepheight1/1
  RegressionData2KeyEvents/1 -> KneeFlexionStepheight/1
  Gain3/1 -> KneeFlexionStepheight/2
  Gain4/1 -> KneeFlexionStepheight1/2
  StepHeight_KneeFlexion_pct/1 -> Gain4/1, Gain3/1
  HipExtensionOffset_pct/1 -> GainHipExtensionOffset/1
  KneeFlexionStepheight1/1 -> AddToMatrixColumn/1
  GainHipExtensionOffset/1 -> AddToMatrixColumn/2
  RatioFlexionExtension/1 -> Bias1/1
  MultiplyMatrixElement/1 -> MultiplyMatrixElement2/1
  MultiplyMatrixElement2/1 -> MultiplyMatrixElement3/1
  MultiplyMatrixElement3/1 -> MultiplyMatrixElement1/1
